simulink model "ps_2016"  (R2016b)
settings: Solver=ode23tb  StartTime=0.0  StopTime=0.6  RelTol=1e-3
libraries: powerlib x34, re_lib x6, powerlib_meascontrol x3
settings Model: Creator=Muhi zatar  LastModifiedBy=Muhi zatar
settings SimscapeCC: SimscapeNormalizeSystem=off

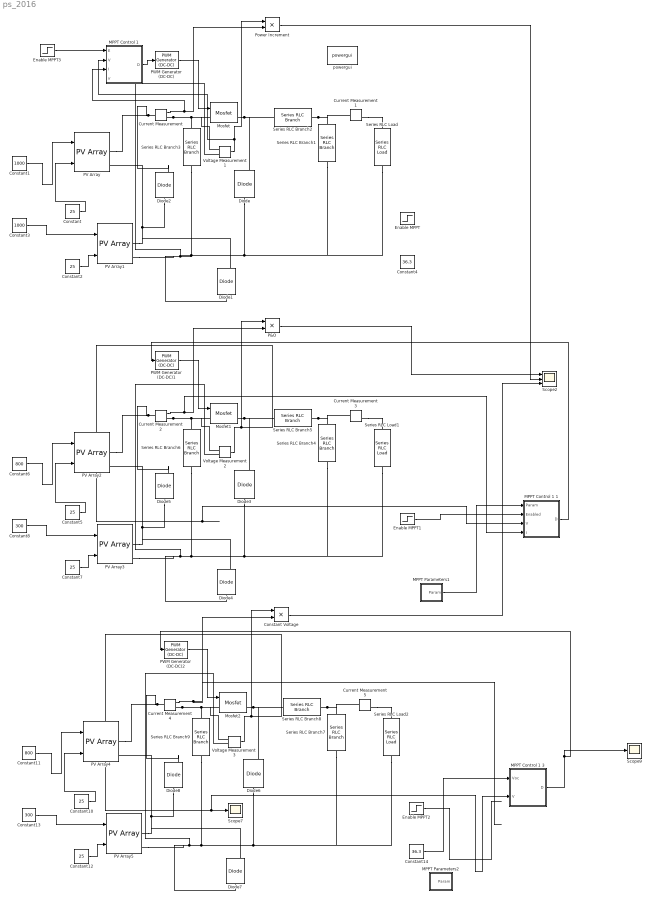
== system ps_2016 ==
  Constant{,2,5,7,10,12} (6 alike) : Constant  Value=25
  Constant Voltage : Product
  Constant1 : Constant  Value=1000
  Constant11 : Constant  Value=800
  Constant13 : Constant  Value=300
  Constant14 : Constant  Value=36.3
  Constant3 : Constant  Value=1000
  Constant4 : Constant  Value=36.3
  Constant6 : Constant  Value=800
  Constant8 : Constant  Value=300
  Current Measurement{,1..5} (6 alike) : powerlib/Measurements/Current Measurement  PhasorSimulation=off  OutputType=Complex  PSBequivalent=0
  Diode : powerlib/Power Electronics/Diode  Ron=0.000001  Lon=0  Vf=0  IC=0  UseSnubber=off  Rs=500  Cs=250e-9  Measurements=on
  Diode{1..2,4..5,7..8} (6 alike) : powerlib/Power Electronics/Diode  Ron=0.001  Lon=0  Vf=0  IC=0  UseSnubber=off  Rs=1e5*inf  Cs=inf  Measurements=on
  Diode3 : powerlib/Power Electronics/Diode  Ron=0.000001  Lon=0  Vf=0  IC=0  UseSnubber=off  Rs=500  Cs=250e-9  Measurements=on
  Diode6 : powerlib/Power Electronics/Diode  Ron=0.000001  Lon=0  Vf=0  IC=0  UseSnubber=off  Rs=500  Cs=250e-9  Measurements=on
  Enable MPPT : Step  Time=0.01  SampleTime=0
  Enable MPPT1 : Step  Time=0  SampleTime=0
  Enable MPPT2 : Step  Time=0  SampleTime=0
  Enable MPPT3 : Step  Time=0  SampleTime=0
  MPPT Parameters1 : Subsystem
  MPPT Parameters2 : Subsystem
  "MPPT Control 1 " : MATLAB Function  TreatAsAtomicUnit=on
  MPPT Control 1 1 : MATLAB Function  TreatAsAtomicUnit=on
  MPPT Control 1 3 : MATLAB Function  TreatAsAtomicUnit=on
  Mosfet : powerlib/Power Electronics/Mosfet  Ron=0.0000001  Lon=0  Rd=0.0000001  Vfd=0  IC=0  Rs=1e5  Cs=inf  Measurements=on
  Mosfet1 : powerlib/Power Electronics/Mosfet  Ron=0.0000001  Lon=0  Rd=0.0000001  Vfd=0  IC=0  Rs=1e5  Cs=inf  Measurements=on
  Mosfet2 : powerlib/Power Electronics/Mosfet  Ron=0.0000001  Lon=0  Rd=0.0000001  Vfd=0  IC=0  Rs=1e5  Cs=inf  Measurements=on
  P&O : Product
  PV Array{,1..5} (6 alike) : re_lib/Solar/PV Array  Npar=1  Nser=1  PlotType=array @ 25 deg.C & specified irradiances  S_vec="[ 1000  800  500 ]"  Temp_C_vec="[ 45 25  ]"  ModuleName=User-defined  PlotWhenSelected=off  Pm=106.575  Ncell=60  Voc=18.15  Isc=7.84  Vm=14.5  Im=7.35  beta_Voc_pc=-0.36099  alpha_Isc_pc=0.102  beta_Voc=-0.06552  alpha_Isc=0.0079968  IL=7.8525  I0=2.8967e-10  nI=0.49035  Rsh=195.9636  Rs=0.19711  BAL=off  Tc=1e-6  Tfilter=5e-5
  PWM Generator (DC-DC) : powerlib_meascontrol/Pulse & Signal Generators/PWM Generator (DC-DC)  Fsw=50000  Ts=0
  PWM Generator (DC-DC)1 : powerlib_meascontrol/Pulse & Signal Generators/PWM Generator (DC-DC)  Fsw=50000  Ts=0
  PWM Generator (DC-DC)2 : powerlib_meascontrol/Pulse & Signal Generators/PWM Generator (DC-DC)  Fsw=50000  Ts=0
  Power Increment : Product
  Scope2 : Scope  NumInputPorts=3
  Scope7 : Scope
  Scope9 : Scope
  Series RLC Branch1 : powerlib/Elements/Series RLC Branch  LConnTagsString=__new0  RConnTagsString=__new0  BranchType=C  Resistance=0.01  Inductance=1e-3  SetiL0=off  InitialCurrent=0  Capacitance=1e-3  Setx0=off  InitialVoltage=0  Measurements=None
  Series RLC Branch2 : powerlib/Elements/Series RLC Branch  LConnTagsString=__new0  RConnTagsString=__new0  BranchType=L  Resistance=5  Inductance=1e-3  SetiL0=off  InitialCurrent=0  Capacitance=1e-6  Setx0=off  InitialVoltage=0  Measurements=None
  Series RLC Branch3 : powerlib/Elements/Series RLC Branch  LConnTagsString=__new0  RConnTagsString=__new0  BranchType=C  Resistance=5  Inductance=1e-3  SetiL0=off  InitialCurrent=0  Capacitance=1e-3  Setx0=off  InitialVoltage=0  Measurements=None
  Series RLC Branch4 : powerlib/Elements/Series RLC Branch  LConnTagsString=__new0  RConnTagsString=__new0  BranchType=C  Resistance=0.01  Inductance=1e-3  SetiL0=off  InitialCurrent=0  Capacitance=1e-3  Setx0=off  InitialVoltage=0  Measurements=None
  Series RLC Branch5 : powerlib/Elements/Series RLC Branch  LConnTagsString=__new0  RConnTagsString=__new0  BranchType=L  Resistance=5  Inductance=1e-3  SetiL0=off  InitialCurrent=0  Capacitance=1e-6  Setx0=off  InitialVoltage=0  Measurements=None
  Series RLC Branch6 : powerlib/Elements/Series RLC Branch  LConnTagsString=__new0  RConnTagsString=__new0  BranchType=C  Resistance=5  Inductance=1e-3  SetiL0=off  InitialCurrent=0  Capacitance=1e-3  Setx0=off  InitialVoltage=0  Measurements=None
  Series RLC Branch7 : powerlib/Elements/Series RLC Branch  LConnTagsString=__new0  RConnTagsString=__new0  BranchType=C  Resistance=0.01  Inductance=1e-3  SetiL0=off  InitialCurrent=0  Capacitance=1e-3  Setx0=off  InitialVoltage=0  Measurements=None
  Series RLC Branch8 : powerlib/Elements/Series RLC Branch  LConnTagsString=__new0  RConnTagsString=__new0  BranchType=L  Resistance=5  Inductance=1e-3  SetiL0=off  InitialCurrent=0  Capacitance=1e-6  Setx0=off  InitialVoltage=0  Measurements=None
  Series RLC Branch9 : powerlib/Elements/Series RLC Branch  LConnTagsString=__new0  RConnTagsString=__new0  BranchType=C  Resistance=5  Inductance=1e-3  SetiL0=off  InitialCurrent=0  Capacitance=1e-3  Setx0=off  InitialVoltage=0  Measurements=None
  Series RLC Load : powerlib/Elements/Series RLC Load  LConnTagsString=a  RConnTagsString=__new0  NominalVoltage=10  NominalFrequency=60  ActivePower=210  InductivePower=0  CapacitivePower=0  Setx0=off  InitialVoltage=0  SetiL0=off  InitialCurrent=0  Measurements=None  LoadType=constant Z
  Series RLC Load1 : powerlib/Elements/Series RLC Load  LConnTagsString=a  RConnTagsString=__new0  NominalVoltage=10  NominalFrequency=60  ActivePower=210  InductivePower=0  CapacitivePower=0  Setx0=off  InitialVoltage=0  SetiL0=off  InitialCurrent=0  Measurements=None  LoadType=constant Z
  Series RLC Load2 : powerlib/Elements/Series RLC Load  LConnTagsString=a  RConnTagsString=__new0  NominalVoltage=10  NominalFrequency=60  ActivePower=210  InductivePower=0  CapacitivePower=0  Setx0=off  InitialVoltage=0  SetiL0=off  InitialCurrent=0  Measurements=None  LoadType=constant Z
  Voltage Measurement1 : powerlib/Measurements/Voltage Measurement  PhasorSimulation=off  OutputType=Complex  PSBequivalent=0
  Voltage Measurement2 : powerlib/Measurements/Voltage Measurement  PhasorSimulation=off  OutputType=Complex  PSBequivalent=0
  Voltage Measurement3 : powerlib/Measurements/Voltage Measurement  PhasorSimulation=off  OutputType=Complex  PSBequivalent=0
  powergui : powerlib/powergui  Priority=1  SimulationMode=Discrete  SampleTime=1e-7  frequency=60  Iterations=50  frequencyindice=0  Pbase=100e6  ErrMax=1e-4  UnitsV=kV  UnitsW=MW  buscounter=0  FunctionMessages=off  echomessages=off  EnableUseOfTLC=off  CurrentSourceSwitches=off  DisableSnubberDevices=off  DisableRonSwitches=off  DisableVfSwitches=off  DisplayEquations=off  SolverType=Tustin/Backward Euler (TBE)  Interpol=off  ExternalGateDelay=off  methode=off  Ts=10  x0status=blocks  SPID=off  SwTol=0  HookPort=off  RestoreLinks=warning  ResistiveCurrentMeasurement=off  Frange=[0:2:500]  Ylog=off  Xlog=on  ShowGrid=off  save=off  variable=ZData  structure=0  ZoomFFT=off  StartTime=0.0  cycles=1  DisplayStyle=1  fundamental=60  FreqAxis=off  MaxFrequency=1000  frequencyindicesteady=1  RmsSteady=1  display=off
  wires:
  Constant1/1 -> PV Array/1
  Constant/1 -> PV Array/2
  Current Measurement/1 -> "MPPT Control 1 "/3(I), Power Increment/2
  PWM Generator (DC-DC)/1 -> Mosfet/1
  Voltage Measurement1/1 -> "MPPT Control 1 "/2(V), Power Increment/1
  Power Increment/1 -> Scope2/2
  Constant2/1 -> PV Array1/2
  Constant3/1 -> PV Array1/1
  Constant6/1 -> PV Array2/1
  Constant5/1 -> PV Array2/2
  Current Measurement2/1 -> MPPT Control 1 1/4(I), P&O/2
  PWM Generator (DC-DC)1/1 -> Mosfet1/1
  Voltage Measurement2/1 -> P&O/1, MPPT Control 1 1/3(V)
  P&O/1 -> Scope2/1
  MPPT Control 1 1/1(D) -> PWM Generator (DC-DC)1/1
  Constant7/1 -> PV Array3/2
  Constant8/1 -> PV Array3/1
  Enable MPPT1/1 -> MPPT Control 1 1/2(Enabled)
  ? -> ?
  Constant11/1 -> PV Array4/1
  Constant10/1 -> PV Array4/2
  Current Measurement4/1 -> Constant Voltage/2
  PWM Generator (DC-DC)2/1 -> Mosfet2/1
  Voltage Measurement3/1 -> Constant Voltage/1, MPPT Control 1 3/2(V), Scope7/1
  Constant Voltage/1 -> Scope2/3
  MPPT Control 1 3/1(D) -> PWM Generator (DC-DC)2/1, Scope9/1
  Constant12/1 -> PV Array5/2
  Constant13/1 -> PV Array5/1
  Enable MPPT2/1 -> ?
  Constant14/1 -> MPPT Control 1 3/1(Voc)
  MPPT Parameters1/1(Param) -> MPPT Control 1 1/1(Param)
  "MPPT Control 1 "/1(D) -> PWM Generator (DC-DC)/1
  Enable MPPT3/1 -> "MPPT Control 1 "/1(E)
  connections:
  Current Measurement/RConn1 -- Series RLC Branch3/LConn1 -- Voltage Measurement1/LConn1 -- Mosfet/LConn1
  Mosfet/RConn1 -- Series RLC Branch2/LConn1 -- Diode/RConn1
  Series RLC Branch3/RConn1 -- Series RLC Load/RConn1 -- Series RLC Branch1/RConn1 -- Diode/LConn1 -- Voltage Measurement1/LConn2 -- PV Array1/RConn2 -- Diode1/LConn1
  Series RLC Branch2/RConn1 -- Current Measurement1/LConn1 -- Series RLC Branch1/LConn1
  Diode2/LConn1 -- PV Array/RConn2 -- PV Array1/RConn1 -- Diode1/RConn1
  Current Measurement/LConn1 -- PV Array/RConn1 -- Diode2/RConn1
  Current Measurement1/RConn1 -- Series RLC Load/LConn1
  Current Measurement2/RConn1 -- Series RLC Branch6/LConn1 -- Voltage Measurement2/LConn1 -- Mosfet1/LConn1
  Mosfet1/RConn1 -- Series RLC Branch5/LConn1 -- Diode3/RConn1
  Series RLC Branch6/RConn1 -- Series RLC Load1/RConn1 -- Series RLC Branch4/RConn1 -- Diode3/LConn1 -- Voltage Measurement2/LConn2 -- PV Array3/RConn2 -- Diode4/LConn1
  Series RLC Branch5/RConn1 -- Current Measurement3/LConn1 -- Series RLC Branch4/LConn1
  Diode5/LConn1 -- PV Array2/RConn2 -- PV Array3/RConn1 -- Diode4/RConn1
  Current Measurement2/LConn1 -- PV Array2/RConn1 -- Diode5/RConn1
  Current Measurement3/RConn1 -- Series RLC Load1/LConn1
  Current Measurement4/RConn1 -- Series RLC Branch9/LConn1 -- Voltage Measurement3/LConn1 -- Mosfet2/LConn1
  Mosfet2/RConn1 -- Series RLC Branch8/LConn1 -- Diode6/RConn1
  Series RLC Branch9/RConn1 -- Series RLC Load2/RConn1 -- Series RLC Branch7/RConn1 -- Diode6/LConn1 -- Voltage Measurement3/LConn2 -- PV Array5/RConn2 -- Diode7/LConn1
  Series RLC Branch8/RConn1 -- Current Measurement5/LConn1 -- Series RLC Branch7/LConn1
  Diode8/LConn1 -- PV Array4/RConn2 -- PV Array5/RConn1 -- Diode7/RConn1
  Current Measurement4/LConn1 -- PV Array4/RConn1 -- Diode8/RConn1
  Current Measurement5/RConn1 -- Series RLC Load2/LConn1

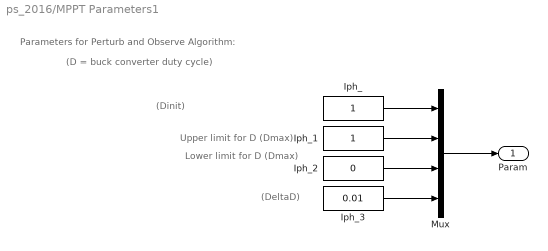
== system ps_2016/MPPT Parameters1 ==
  note: Upper limit for D (Dmax)
  note: (DeltaD)
  note: (Dinit)
  note: (D = buck converter duty cycle)
  note: Lower limit for D (Dmax)
  note: Parameters for Perturb and Observe Algorithm:
  Iph_ : Constant
  Iph_1 : Constant
  Iph_2 : Constant  Value=0
  Iph_3 : Constant  Value=0.01
  Mux : Mux
  Param : Outport
  wires:
  Iph_/1 -> Mux/1
  Iph_1/1 -> Mux/2
  Iph_2/1 -> Mux/3
  Iph_3/1 -> Mux/4
  Mux/1 -> Param/1

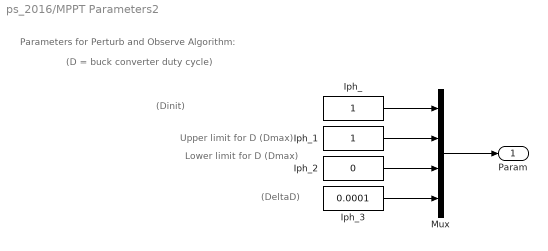
== system ps_2016/MPPT Parameters2 ==
  note: Upper limit for D (Dmax)
  note: (DeltaD)
  note: (Dinit)
  note: (D = buck converter duty cycle)
  note: Lower limit for D (Dmax)
  note: Parameters for Perturb and Observe Algorithm:
  Iph_ : Constant
  Iph_1 : Constant
  Iph_2 : Constant  Value=0
  Iph_3 : Constant  Value=0.0001
  Mux : Mux
  Param : Outport
  wires:
  Iph_/1 -> Mux/1
  Iph_1/1 -> Mux/2
  Iph_2/1 -> Mux/3
  Iph_3/1 -> Mux/4
  Mux/1 -> Param/1

== matlab function ps_2016/MPPT Control 1 1 ==
  settings: updateMethod=DISCRETE  sampleTime=Ts_Control
  data: Param input; Enabled input; V input =V; I input; D output
function D  = PandO(Param, Enabled, V, I)

% MPPT controller based on the Perturb & Observe algorithm.

% D output = Duty cycle of the boost converter (value between 0 and 1)
%
% Enabled input = 1 to enable the MPPT controller
% V input = PV array terminal voltage (V)
% I input = PV array current (A)
%
% Param input:
Dinit = Param(1);  %Initial value for D output
Dmax = Param(2);   %Maximum value for D
Dmin = Param(3);   %Minimum value for D
deltaD = Param(4); %Increment value used to increase/decrease the duty cycle D
% ( increasing D = decreasing Vref )
%  

persistent Vold Pold Dold;

dataType = 'double';

if isempty(Vold)
    Vold=0;
    Pold=0;
    Dold=Dinit;
end
P= V*I;
dV= V - Vold;
dP= P - Pold;

if dP ~= 0 & Enabled ~=0
    if dP < 0
        if dV < 0
            D = Dold - deltaD;
        else
            D = Dold + deltaD;
        end
    else
        if dV < 0
            D = Dold + deltaD;
        else
            D = Dold - deltaD;
        end    
    end
else D=Dold;
end

if D >= Dmax | D<= Dmin
    D=Dold;
end

Dold=D;
Vold=V;
Pold=P;

== matlab function ps_2016/MPPT Control 1 3 ==
  settings: updateMethod=DISCRETE  sampleTime=Ts_Control
  data: Voc input; V input =V; D output
function D  = PandO(Voc, V)
persistent Dold1 ;
dataType = 'double';
if isempty(Dold1)
    Dold1=0.3;
end

Vmax=0.85*Voc;
Vmin=0.75*Voc;

if V>Vmin && V<Vmax 
    D=Dold1;
    
else
    if V>Vmax 
        D=Dold1+0.0008;
    else
        D = Dold1-0.0008;
    end
end
Dold1=D;

end

== matlab function ps_2016/MPPT Control 1  ==
  settings: updateMethod=DISCRETE  sampleTime=Ts_Control
  data: E input; V input =V; I input; D output; ir input
function D  = powerincrement(E,V, I,ir)
persistent Pold;
persistent Dold;
persistent Pnow;
persistent Dmax;
persistent P;
persistent Pmax;
persistent irold;
dataType = 'double';
if isempty(irold)
    irold=0;
end
if isempty(Dold)
    Dold=0.9;
end
if isempty(Pmax)
    Pmax=0;
end
if isempty(P)
    P=0;
end
if isempty(Dmax)
    Dmax=0.9;
end
if isempty(Pold)
    Pold=0;
end
if irold-ir>5
    Dold=0.9;
    Pmax=0;
    Pold=0;
    Dmax=0.9;
end
Pnow = I*V;
if Pnow>Pold  && E~=0 && Dold>0
    Dmax=Dold;
    Pold=Pnow;
end

if Dold>0 && E~=0 && Dold>0
    Dold=Dold-0.0003;
end

if Dold>0 && E~=0
    D=Dold;
else
    D=Dmax;
end

irold=ir;
